simulink model "rezervor_cu_perturbatie"  (R2022b)
settings: Solver=VariableStepAuto  StartTime=0.0  StopTime=10.0  RelTol=1e-3
values from neighbouring files (symbols this model uses):
  A = 332.5    [run_first.m]
  C = 8.45    [run_first.m]
settings Model: Creator=fabian  LastModifiedBy=fabian

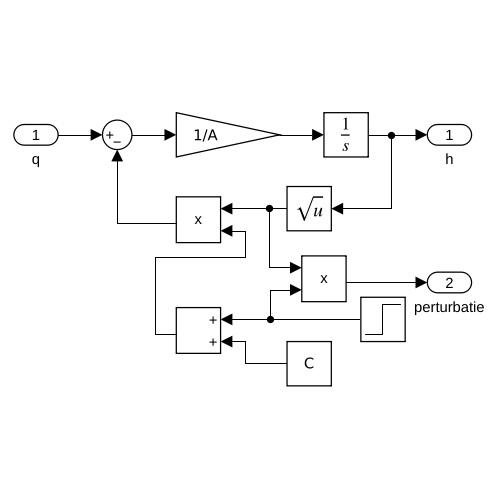
[thumbnail: Simulink's stored preview of the top-level diagram]
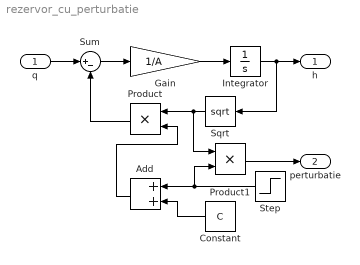
== system rezervor_cu_perturbatie ==
  q : Inport
  Add : Sum
  Constant : Constant  Value=C
  Gain : Gain  Gain=1/A
  Integrator : Integrator  InitialCondition=16.9
  Product : Product
  Product1 : Product
  Sqrt : Sqrt
  Step : Step  Time=1000  After=0.01  SampleTime=0
  Sum : Sum  Inputs=|+-
  h : Outport
  perturbatie : Outport  Port=2
  wires:
  q/1 -> Sum/1
  Product/1 -> Sum/2
  Sum/1 -> Gain/1
  Gain/1 -> Integrator/1
  Integrator/1 -> Sqrt/1, h/1
  Sqrt/1 -> Product1/1, Product/1
  Step/1 -> Product1/2, Add/1
  Product1/1 -> perturbatie/1
  Add/1 -> Product/2
  Constant/1 -> Add/2
